simulink model "receiver_overall_reset"  (Simulink 7.5)
settings: Solver=FixedStepDiscrete  SolverMode=SingleTasking  StartTime=0.0  StopTime=(length(simin.signals.values)-1)/Fs  FixedStep=1  RelTol=1e-3
undefined symbols (not defined in the file): Fs
libraries: xbsIndex_r4 x962
(part 5 of 9)

== system receiver_overall_reset/Receiver/Sym-Chooser/2-10/Corr0/Corr ==
  In1 : Inport
  AddSub{,1..6} (7 alike) : xbsIndex_r4/AddSub  mode=Addition  use_carryin=off  use_carryout=off  en=off  latency=0  precision=Full  arith_type=Unsigned  n_bits=16  bin_pt=14  quantization=Truncate  overflow=Wrap  dbl_ovrd=off  use_behavioral_HDL=off  hw_selection=Fabric  pipelined=off  block_type=addsub
      AddSub settings: xl_area=[2 0 0 3 0 0 0]  block_version=12.1
      AddSub1 settings: xl_area=[2 0 0 3 0 0 0]  block_version=12.1
      AddSub2 settings: xl_area=[3 0 0 4 0 0 0]  block_version=12.1
      AddSub3 settings: xl_area=[3 0 0 5 0 0 0]  block_version=12.1
      AddSub4 settings: xl_area=[2 0 0 3 0 0 0]  block_version=12.1
      AddSub5 settings: xl_area=[2 0 0 3 0 0 0]  block_version=12.1
      AddSub6 settings: xl_area=[3 0 0 4 0 0 0]  block_version=12.1
  LUT{0..7} (8 alike) : xbsIndex_r4/ROM  depth=16  initVector=[0,1,1,2,1,2,2,3,1,2,2,3,2,3,3,4]  distributed_mem=Distributed memory  rst=off  init_reg=0  en=off  latency=0  arith_type=Unsigned  n_bits=3  bin_pt=0  dbl_ovrd=off  optimize=Area  use_rpm=on  block_type=sprom
      settings: xl_area=[0 0 1 0 0 0 0]  block_version=12.1
  Slice0 : xbsIndex_r4/Slice  nbits=4  boolean_output=off  mode=Lower Bit Location + Width  bit1=0  base1=MSB of Input  bit0=0  base0=LSB of Input  dbl_ovrd=off  block_type=slice
      settings: block_version=12.1
  Slice1 : xbsIndex_r4/Slice  nbits=4  boolean_output=off  mode=Lower Bit Location + Width  bit1=-4  base1=MSB of Input  bit0=4  base0=LSB of Input  dbl_ovrd=off  block_type=slice
      settings: block_version=12.1
  Slice2 : xbsIndex_r4/Slice  nbits=4  boolean_output=off  mode=Lower Bit Location + Width  bit1=-8  base1=MSB of Input  bit0=8  base0=LSB of Input  dbl_ovrd=off  block_type=slice
      settings: block_version=12.1
  Slice3 : xbsIndex_r4/Slice  nbits=4  boolean_output=off  mode=Lower Bit Location + Width  bit1=-12  base1=MSB of Input  bit0=12  base0=LSB of Input  dbl_ovrd=off  block_type=slice
      settings: block_version=12.1
  Slice4 : xbsIndex_r4/Slice  nbits=4  boolean_output=off  mode=Lower Bit Location + Width  bit1=0  base1=LSB of Input  bit0=16  base0=LSB of Input  dbl_ovrd=off  block_type=slice
      settings: block_version=12.1
  Slice5 : xbsIndex_r4/Slice  nbits=4  boolean_output=off  mode=Lower Bit Location + Width  bit1=0  base1=LSB of Input  bit0=20  base0=LSB of Input  dbl_ovrd=off  block_type=slice
      settings: block_version=12.1
  Slice6 : xbsIndex_r4/Slice  nbits=4  boolean_output=off  mode=Lower Bit Location + Width  bit1=0  base1=LSB of Input  bit0=24  base0=LSB of Input  dbl_ovrd=off  block_type=slice
      settings: block_version=12.1
  Slice7 : xbsIndex_r4/Slice  nbits=4  boolean_output=off  mode=Lower Bit Location + Width  bit1=0  base1=LSB of Input  bit0=28  base0=LSB of Input  dbl_ovrd=off  block_type=slice
      settings: block_version=12.1
  Out2 : Outport
  wires:
  In1/1 -> Slice0/1, Slice1/1, Slice2/1, Slice7/1, Slice6/1, Slice3/1, Slice4/1, Slice5/1
  Slice0/1 -> LUT0/1
  Slice3/1 -> LUT3/1
  Slice2/1 -> LUT2/1
  Slice1/1 -> LUT1/1
  LUT0/1 -> AddSub/1
  LUT1/1 -> AddSub/2
  LUT2/1 -> AddSub1/1
  LUT3/1 -> AddSub1/2
  AddSub1/1 -> AddSub2/2
  AddSub/1 -> AddSub2/1
  AddSub3/1 -> Out2/1
  Slice4/1 -> LUT4/1
  Slice7/1 -> LUT7/1
  Slice6/1 -> LUT6/1
  Slice5/1 -> LUT5/1
  LUT4/1 -> AddSub4/1
  LUT5/1 -> AddSub4/2
  LUT6/1 -> AddSub5/1
  LUT7/1 -> AddSub5/2
  AddSub5/1 -> AddSub6/2
  AddSub4/1 -> AddSub6/1
  AddSub2/1 -> AddSub3/1
  AddSub6/1 -> AddSub3/2

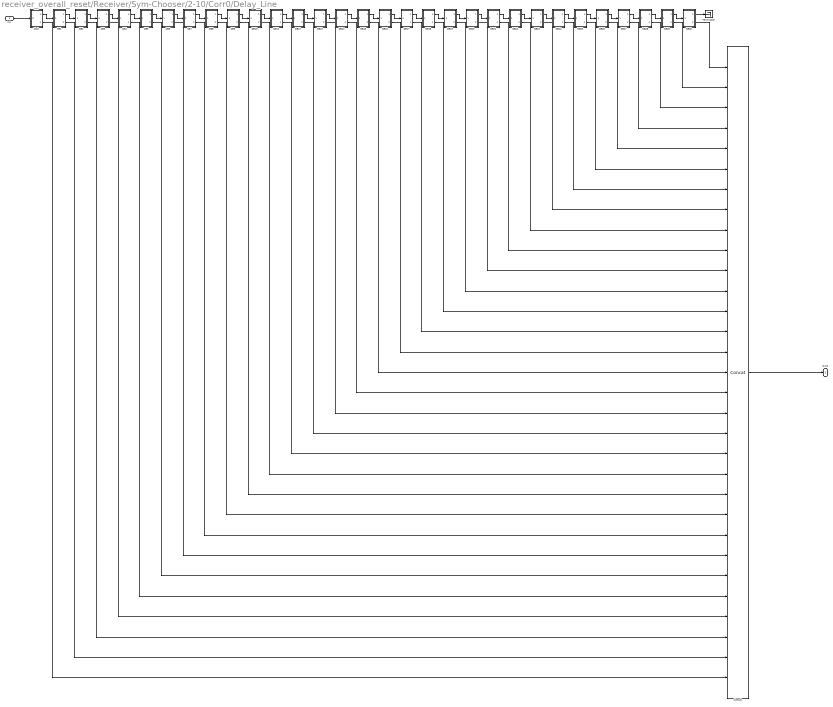
== system receiver_overall_reset/Receiver/Sym-Chooser/2-10/Corr0/Delay_Line ==
  In1 : Inport
  1to2 : Subsystem
  Concat : xbsIndex_r4/Concat  num_inputs=31  dbl_ovrd=off  block_type=concat
      settings: block_version=12.1
  DE1 : Subsystem
      mask Display: disp('z^{-1}','texmode','on')
  DE10 : Subsystem
      mask Display: disp('z^{-1}','texmode','on')
  DE11 : Subsystem
      mask Display: disp('z^{-1}','texmode','on')
  DE12 : Subsystem
      mask Display: disp('z^{-1}','texmode','on')
  DE13 : Subsystem
      mask Display: disp('z^{-1}','texmode','on')
  DE14 : Subsystem
      mask Display: disp('z^{-1}','texmode','on')
  DE15 : Subsystem
      mask Display: disp('z^{-1}','texmode','on')
  DE16 : Subsystem
      mask Display: disp('z^{-1}','texmode','on')
  DE17 : Subsystem
      mask Display: disp('z^{-1}','texmode','on')
  DE18 : Subsystem
      mask Display: disp('z^{-1}','texmode','on')
  DE19 : Subsystem
      mask Display: disp('z^{-1}','texmode','on')
  DE2 : Subsystem
      mask Display: disp('z^{-1}','texmode','on')
  DE20 : Subsystem
      mask Display: disp('z^{-1}','texmode','on')
  DE21 : Subsystem
      mask Display: disp('z^{-1}','texmode','on')
  DE22 : Subsystem
      mask Display: disp('z^{-1}','texmode','on')
  DE23 : Subsystem
      mask Display: disp('z^{-1}','texmode','on')
  DE24 : Subsystem
      mask Display: disp('z^{-1}','texmode','on')
  DE25 : Subsystem
      mask Display: disp('z^{-1}','texmode','on')
  DE26 : Subsystem
      mask Display: disp('z^{-1}','texmode','on')
  DE27 : Subsystem
      mask Display: disp('z^{-1}','texmode','on')
  DE28 : Subsystem
      mask Display: disp('z^{-1}','texmode','on')
  DE29 : Subsystem
      mask Display: disp('z^{-1}','texmode','on')
  DE3 : Subsystem
      mask Display: disp('z^{-1}','texmode','on')
  DE30 : Subsystem
      mask Display: disp('z^{-1}','texmode','on')
  DE4 : Subsystem
      mask Display: disp('z^{-1}','texmode','on')
  DE5 : Subsystem
      mask Display: disp('z^{-1}','texmode','on')
  DE6 : Subsystem
      mask Display: disp('z^{-1}','texmode','on')
  DE7 : Subsystem
      mask Display: disp('z^{-1}','texmode','on')
  DE8 : Subsystem
      mask Display: disp('z^{-1}','texmode','on')
  DE9 : Subsystem
      mask Display: disp('z^{-1}','texmode','on')
  Terminator : Terminator
  Out2 : Outport
  wires:
  Concat/1 -> Out2/1
  In1/1 -> 1to2/1(In)
  1to2/1(Out1) -> DE1/1(In1)
  DE30/1(Out1) -> Terminator/1
  1to2/2(Out2) -> Concat/31
  DE1/2(Out2) -> Concat/30
  DE2/2(Out2) -> Concat/29
  DE3/2(Out2) -> Concat/28
  DE4/2(Out2) -> Concat/27
  DE5/2(Out2) -> Concat/26
  DE6/2(Out2) -> Concat/25
  DE7/2(Out2) -> Concat/24
  DE8/2(Out2) -> Concat/23
  DE9/2(Out2) -> Concat/22
  DE10/2(Out2) -> Concat/21
  DE11/2(Out2) -> Concat/20
  DE12/2(Out2) -> Concat/19
  DE13/2(Out2) -> Concat/18
  DE14/2(Out2) -> Concat/17
  DE15/2(Out2) -> Concat/16
  DE16/2(Out2) -> Concat/15
  DE17/2(Out2) -> Concat/14
  DE18/2(Out2) -> Concat/13
  DE19/2(Out2) -> Concat/12
  DE20/2(Out2) -> Concat/11
  DE21/2(Out2) -> Concat/10
  DE22/2(Out2) -> Concat/9
  DE23/2(Out2) -> Concat/8
  DE24/2(Out2) -> Concat/7
  DE25/2(Out2) -> Concat/6
  DE26/2(Out2) -> Concat/5
  DE27/2(Out2) -> Concat/4
  DE28/2(Out2) -> Concat/3
  DE29/2(Out2) -> Concat/2
  DE30/2(Out2) -> Concat/1
  DE2/1(Out1) -> DE3/1(In1)
  DE3/1(Out1) -> DE4/1(In1)
  DE4/1(Out1) -> DE5/1(In1)
  DE5/1(Out1) -> DE6/1(In1)
  DE6/1(Out1) -> DE7/1(In1)
  DE7/1(Out1) -> DE8/1(In1)
  DE8/1(Out1) -> DE9/1(In1)
  DE9/1(Out1) -> DE10/1(In1)
  DE10/1(Out1) -> DE11/1(In1)
  DE11/1(Out1) -> DE12/1(In1)
  DE12/1(Out1) -> DE13/1(In1)
  DE13/1(Out1) -> DE14/1(In1)
  DE14/1(Out1) -> DE15/1(In1)
  DE15/1(Out1) -> DE16/1(In1)
  DE16/1(Out1) -> DE17/1(In1)
  DE17/1(Out1) -> DE18/1(In1)
  DE18/1(Out1) -> DE19/1(In1)
  DE19/1(Out1) -> DE20/1(In1)
  DE20/1(Out1) -> DE21/1(In1)
  DE21/1(Out1) -> DE22/1(In1)
  DE22/1(Out1) -> DE23/1(In1)
  DE23/1(Out1) -> DE24/1(In1)
  DE24/1(Out1) -> DE25/1(In1)
  DE25/1(Out1) -> DE26/1(In1)
  DE26/1(Out1) -> DE27/1(In1)
  DE27/1(Out1) -> DE28/1(In1)
  DE28/1(Out1) -> DE29/1(In1)
  DE29/1(Out1) -> DE30/1(In1)
  DE1/1(Out1) -> DE2/1(In1)

== system receiver_overall_reset/Receiver/Sym-Chooser/3-11/Corr0/Corr ==
  In1 : Inport
  AddSub{,1..6} (7 alike) : xbsIndex_r4/AddSub  mode=Addition  use_carryin=off  use_carryout=off  en=off  latency=0  precision=Full  arith_type=Unsigned  n_bits=16  bin_pt=14  quantization=Truncate  overflow=Wrap  dbl_ovrd=off  use_behavioral_HDL=off  hw_selection=Fabric  pipelined=off  block_type=addsub
      AddSub settings: xl_area=[2 0 0 3 0 0 0]  block_version=12.1
      AddSub1 settings: xl_area=[2 0 0 3 0 0 0]  block_version=12.1
      AddSub2 settings: xl_area=[3 0 0 4 0 0 0]  block_version=12.1
      AddSub3 settings: xl_area=[3 0 0 5 0 0 0]  block_version=12.1
      AddSub4 settings: xl_area=[2 0 0 3 0 0 0]  block_version=12.1
      AddSub5 settings: xl_area=[2 0 0 3 0 0 0]  block_version=12.1
      AddSub6 settings: xl_area=[3 0 0 4 0 0 0]  block_version=12.1
  LUT{0..7} (8 alike) : xbsIndex_r4/ROM  depth=16  initVector=[0,1,1,2,1,2,2,3,1,2,2,3,2,3,3,4]  distributed_mem=Distributed memory  rst=off  init_reg=0  en=off  latency=0  arith_type=Unsigned  n_bits=3  bin_pt=0  dbl_ovrd=off  optimize=Area  use_rpm=on  block_type=sprom
      settings: xl_area=[0 0 1 0 0 0 0]  block_version=12.1
  Slice0 : xbsIndex_r4/Slice  nbits=4  boolean_output=off  mode=Lower Bit Location + Width  bit1=0  base1=MSB of Input  bit0=0  base0=LSB of Input  dbl_ovrd=off  block_type=slice
      settings: block_version=12.1
  Slice1 : xbsIndex_r4/Slice  nbits=4  boolean_output=off  mode=Lower Bit Location + Width  bit1=-4  base1=MSB of Input  bit0=4  base0=LSB of Input  dbl_ovrd=off  block_type=slice
      settings: block_version=12.1
  Slice2 : xbsIndex_r4/Slice  nbits=4  boolean_output=off  mode=Lower Bit Location + Width  bit1=-8  base1=MSB of Input  bit0=8  base0=LSB of Input  dbl_ovrd=off  block_type=slice
      settings: block_version=12.1
  Slice3 : xbsIndex_r4/Slice  nbits=4  boolean_output=off  mode=Lower Bit Location + Width  bit1=-12  base1=MSB of Input  bit0=12  base0=LSB of Input  dbl_ovrd=off  block_type=slice
      settings: block_version=12.1
  Slice4 : xbsIndex_r4/Slice  nbits=4  boolean_output=off  mode=Lower Bit Location + Width  bit1=0  base1=LSB of Input  bit0=16  base0=LSB of Input  dbl_ovrd=off  block_type=slice
      settings: block_version=12.1
  Slice5 : xbsIndex_r4/Slice  nbits=4  boolean_output=off  mode=Lower Bit Location + Width  bit1=0  base1=LSB of Input  bit0=20  base0=LSB of Input  dbl_ovrd=off  block_type=slice
      settings: block_version=12.1
  Slice6 : xbsIndex_r4/Slice  nbits=4  boolean_output=off  mode=Lower Bit Location + Width  bit1=0  base1=LSB of Input  bit0=24  base0=LSB of Input  dbl_ovrd=off  block_type=slice
      settings: block_version=12.1
  Slice7 : xbsIndex_r4/Slice  nbits=4  boolean_output=off  mode=Lower Bit Location + Width  bit1=0  base1=LSB of Input  bit0=28  base0=LSB of Input  dbl_ovrd=off  block_type=slice
      settings: block_version=12.1
  Out2 : Outport
  wires:
  In1/1 -> Slice0/1, Slice1/1, Slice2/1, Slice7/1, Slice6/1, Slice3/1, Slice4/1, Slice5/1
  Slice0/1 -> LUT0/1
  Slice3/1 -> LUT3/1
  Slice2/1 -> LUT2/1
  Slice1/1 -> LUT1/1
  LUT0/1 -> AddSub/1
  LUT1/1 -> AddSub/2
  LUT2/1 -> AddSub1/1
  LUT3/1 -> AddSub1/2
  AddSub1/1 -> AddSub2/2
  AddSub/1 -> AddSub2/1
  AddSub3/1 -> Out2/1
  Slice4/1 -> LUT4/1
  Slice7/1 -> LUT7/1
  Slice6/1 -> LUT6/1
  Slice5/1 -> LUT5/1
  LUT4/1 -> AddSub4/1
  LUT5/1 -> AddSub4/2
  LUT6/1 -> AddSub5/1
  LUT7/1 -> AddSub5/2
  AddSub5/1 -> AddSub6/2
  AddSub4/1 -> AddSub6/1
  AddSub2/1 -> AddSub3/1
  AddSub6/1 -> AddSub3/2

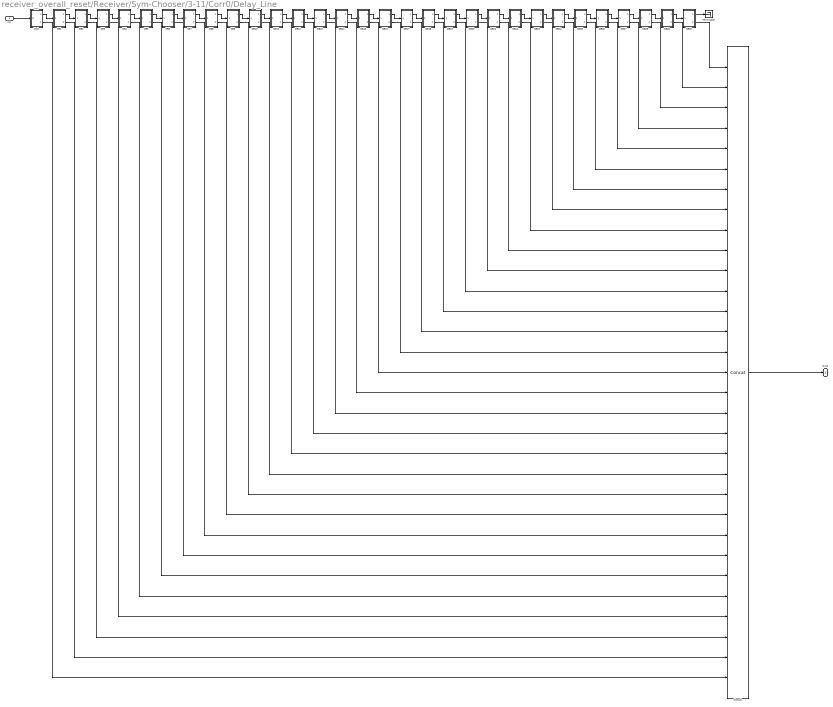
== system receiver_overall_reset/Receiver/Sym-Chooser/3-11/Corr0/Delay_Line ==
  In1 : Inport
  1to2 : Subsystem
  Concat : xbsIndex_r4/Concat  num_inputs=31  dbl_ovrd=off  block_type=concat
      settings: block_version=12.1
  DE1 : Subsystem
      mask Display: disp('z^{-1}','texmode','on')
  DE10 : Subsystem
      mask Display: disp('z^{-1}','texmode','on')
  DE11 : Subsystem
      mask Display: disp('z^{-1}','texmode','on')
  DE12 : Subsystem
      mask Display: disp('z^{-1}','texmode','on')
  DE13 : Subsystem
      mask Display: disp('z^{-1}','texmode','on')
  DE14 : Subsystem
      mask Display: disp('z^{-1}','texmode','on')
  DE15 : Subsystem
      mask Display: disp('z^{-1}','texmode','on')
  DE16 : Subsystem
      mask Display: disp('z^{-1}','texmode','on')
  DE17 : Subsystem
      mask Display: disp('z^{-1}','texmode','on')
  DE18 : Subsystem
      mask Display: disp('z^{-1}','texmode','on')
  DE19 : Subsystem
      mask Display: disp('z^{-1}','texmode','on')
  DE2 : Subsystem
      mask Display: disp('z^{-1}','texmode','on')
  DE20 : Subsystem
      mask Display: disp('z^{-1}','texmode','on')
  DE21 : Subsystem
      mask Display: disp('z^{-1}','texmode','on')
  DE22 : Subsystem
      mask Display: disp('z^{-1}','texmode','on')
  DE23 : Subsystem
      mask Display: disp('z^{-1}','texmode','on')
  DE24 : Subsystem
      mask Display: disp('z^{-1}','texmode','on')
  DE25 : Subsystem
      mask Display: disp('z^{-1}','texmode','on')
  DE26 : Subsystem
      mask Display: disp('z^{-1}','texmode','on')
  DE27 : Subsystem
      mask Display: disp('z^{-1}','texmode','on')
  DE28 : Subsystem
      mask Display: disp('z^{-1}','texmode','on')
  DE29 : Subsystem
      mask Display: disp('z^{-1}','texmode','on')
  DE3 : Subsystem
      mask Display: disp('z^{-1}','texmode','on')
  DE30 : Subsystem
      mask Display: disp('z^{-1}','texmode','on')
  DE4 : Subsystem
      mask Display: disp('z^{-1}','texmode','on')
  DE5 : Subsystem
      mask Display: disp('z^{-1}','texmode','on')
  DE6 : Subsystem
      mask Display: disp('z^{-1}','texmode','on')
  DE7 : Subsystem
      mask Display: disp('z^{-1}','texmode','on')
  DE8 : Subsystem
      mask Display: disp('z^{-1}','texmode','on')
  DE9 : Subsystem
      mask Display: disp('z^{-1}','texmode','on')
  Terminator : Terminator
  Out2 : Outport
  wires:
  Concat/1 -> Out2/1
  In1/1 -> 1to2/1(In)
  1to2/1(Out1) -> DE1/1(In1)
  DE30/1(Out1) -> Terminator/1
  1to2/2(Out2) -> Concat/31
  DE1/2(Out2) -> Concat/30
  DE2/2(Out2) -> Concat/29
  DE3/2(Out2) -> Concat/28
  DE4/2(Out2) -> Concat/27
  DE5/2(Out2) -> Concat/26
  DE6/2(Out2) -> Concat/25
  DE7/2(Out2) -> Concat/24
  DE8/2(Out2) -> Concat/23
  DE9/2(Out2) -> Concat/22
  DE10/2(Out2) -> Concat/21
  DE11/2(Out2) -> Concat/20
  DE12/2(Out2) -> Concat/19
  DE13/2(Out2) -> Concat/18
  DE14/2(Out2) -> Concat/17
  DE15/2(Out2) -> Concat/16
  DE16/2(Out2) -> Concat/15
  DE17/2(Out2) -> Concat/14
  DE18/2(Out2) -> Concat/13
  DE19/2(Out2) -> Concat/12
  DE20/2(Out2) -> Concat/11
  DE21/2(Out2) -> Concat/10
  DE22/2(Out2) -> Concat/9
  DE23/2(Out2) -> Concat/8
  DE24/2(Out2) -> Concat/7
  DE25/2(Out2) -> Concat/6
  DE26/2(Out2) -> Concat/5
  DE27/2(Out2) -> Concat/4
  DE28/2(Out2) -> Concat/3
  DE29/2(Out2) -> Concat/2
  DE30/2(Out2) -> Concat/1
  DE2/1(Out1) -> DE3/1(In1)
  DE3/1(Out1) -> DE4/1(In1)
  DE4/1(Out1) -> DE5/1(In1)
  DE5/1(Out1) -> DE6/1(In1)
  DE6/1(Out1) -> DE7/1(In1)
  DE7/1(Out1) -> DE8/1(In1)
  DE8/1(Out1) -> DE9/1(In1)
  DE9/1(Out1) -> DE10/1(In1)
  DE10/1(Out1) -> DE11/1(In1)
  DE11/1(Out1) -> DE12/1(In1)
  DE12/1(Out1) -> DE13/1(In1)
  DE13/1(Out1) -> DE14/1(In1)
  DE14/1(Out1) -> DE15/1(In1)
  DE15/1(Out1) -> DE16/1(In1)
  DE16/1(Out1) -> DE17/1(In1)
  DE17/1(Out1) -> DE18/1(In1)
  DE18/1(Out1) -> DE19/1(In1)
  DE19/1(Out1) -> DE20/1(In1)
  DE20/1(Out1) -> DE21/1(In1)
  DE21/1(Out1) -> DE22/1(In1)
  DE22/1(Out1) -> DE23/1(In1)
  DE23/1(Out1) -> DE24/1(In1)
  DE24/1(Out1) -> DE25/1(In1)
  DE25/1(Out1) -> DE26/1(In1)
  DE26/1(Out1) -> DE27/1(In1)
  DE27/1(Out1) -> DE28/1(In1)
  DE28/1(Out1) -> DE29/1(In1)
  DE29/1(Out1) -> DE30/1(In1)
  DE1/1(Out1) -> DE2/1(In1)

== system receiver_overall_reset/Receiver/Sym-Chooser/4-12/Corr0/Corr ==
  In1 : Inport
  AddSub{,1..6} (7 alike) : xbsIndex_r4/AddSub  mode=Addition  use_carryin=off  use_carryout=off  en=off  latency=0  precision=Full  arith_type=Unsigned  n_bits=16  bin_pt=14  quantization=Truncate  overflow=Wrap  dbl_ovrd=off  use_behavioral_HDL=off  hw_selection=Fabric  pipelined=off  block_type=addsub
      AddSub settings: xl_area=[2 0 0 3 0 0 0]  block_version=12.1
      AddSub1 settings: xl_area=[2 0 0 3 0 0 0]  block_version=12.1
      AddSub2 settings: xl_area=[3 0 0 4 0 0 0]  block_version=12.1
      AddSub3 settings: xl_area=[3 0 0 5 0 0 0]  block_version=12.1
      AddSub4 settings: xl_area=[2 0 0 3 0 0 0]  block_version=12.1
      AddSub5 settings: xl_area=[2 0 0 3 0 0 0]  block_version=12.1
      AddSub6 settings: xl_area=[3 0 0 4 0 0 0]  block_version=12.1
  LUT{0..7} (8 alike) : xbsIndex_r4/ROM  depth=16  initVector=[0,1,1,2,1,2,2,3,1,2,2,3,2,3,3,4]  distributed_mem=Distributed memory  rst=off  init_reg=0  en=off  latency=0  arith_type=Unsigned  n_bits=3  bin_pt=0  dbl_ovrd=off  optimize=Area  use_rpm=on  block_type=sprom
      settings: xl_area=[0 0 1 0 0 0 0]  block_version=12.1
  Slice0 : xbsIndex_r4/Slice  nbits=4  boolean_output=off  mode=Lower Bit Location + Width  bit1=0  base1=MSB of Input  bit0=0  base0=LSB of Input  dbl_ovrd=off  block_type=slice
      settings: block_version=12.1
  Slice1 : xbsIndex_r4/Slice  nbits=4  boolean_output=off  mode=Lower Bit Location + Width  bit1=-4  base1=MSB of Input  bit0=4  base0=LSB of Input  dbl_ovrd=off  block_type=slice
      settings: block_version=12.1
  Slice2 : xbsIndex_r4/Slice  nbits=4  boolean_output=off  mode=Lower Bit Location + Width  bit1=-8  base1=MSB of Input  bit0=8  base0=LSB of Input  dbl_ovrd=off  block_type=slice
      settings: block_version=12.1
  Slice3 : xbsIndex_r4/Slice  nbits=4  boolean_output=off  mode=Lower Bit Location + Width  bit1=-12  base1=MSB of Input  bit0=12  base0=LSB of Input  dbl_ovrd=off  block_type=slice
      settings: block_version=12.1
  Slice4 : xbsIndex_r4/Slice  nbits=4  boolean_output=off  mode=Lower Bit Location + Width  bit1=0  base1=LSB of Input  bit0=16  base0=LSB of Input  dbl_ovrd=off  block_type=slice
      settings: block_version=12.1
  Slice5 : xbsIndex_r4/Slice  nbits=4  boolean_output=off  mode=Lower Bit Location + Width  bit1=0  base1=LSB of Input  bit0=20  base0=LSB of Input  dbl_ovrd=off  block_type=slice
      settings: block_version=12.1
  Slice6 : xbsIndex_r4/Slice  nbits=4  boolean_output=off  mode=Lower Bit Location + Width  bit1=0  base1=LSB of Input  bit0=24  base0=LSB of Input  dbl_ovrd=off  block_type=slice
      settings: block_version=12.1
  Slice7 : xbsIndex_r4/Slice  nbits=4  boolean_output=off  mode=Lower Bit Location + Width  bit1=0  base1=LSB of Input  bit0=28  base0=LSB of Input  dbl_ovrd=off  block_type=slice
      settings: block_version=12.1
  Out2 : Outport
  wires:
  In1/1 -> Slice0/1, Slice1/1, Slice2/1, Slice7/1, Slice6/1, Slice3/1, Slice4/1, Slice5/1
  Slice0/1 -> LUT0/1
  Slice3/1 -> LUT3/1
  Slice2/1 -> LUT2/1
  Slice1/1 -> LUT1/1
  LUT0/1 -> AddSub/1
  LUT1/1 -> AddSub/2
  LUT2/1 -> AddSub1/1
  LUT3/1 -> AddSub1/2
  AddSub1/1 -> AddSub2/2
  AddSub/1 -> AddSub2/1
  AddSub3/1 -> Out2/1
  Slice4/1 -> LUT4/1
  Slice7/1 -> LUT7/1
  Slice6/1 -> LUT6/1
  Slice5/1 -> LUT5/1
  LUT4/1 -> AddSub4/1
  LUT5/1 -> AddSub4/2
  LUT6/1 -> AddSub5/1
  LUT7/1 -> AddSub5/2
  AddSub5/1 -> AddSub6/2
  AddSub4/1 -> AddSub6/1
  AddSub2/1 -> AddSub3/1
  AddSub6/1 -> AddSub3/2

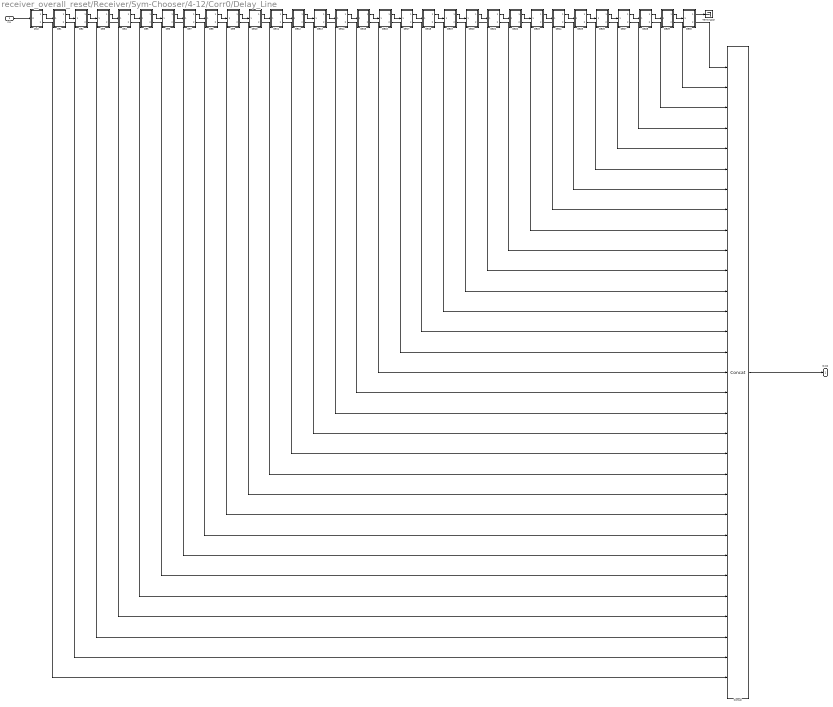
== system receiver_overall_reset/Receiver/Sym-Chooser/4-12/Corr0/Delay_Line ==
  In1 : Inport
  1to2 : Subsystem
  Concat : xbsIndex_r4/Concat  num_inputs=31  dbl_ovrd=off  block_type=concat
      settings: block_version=12.1
  DE1 : Subsystem
      mask Display: disp('z^{-1}','texmode','on')
  DE10 : Subsystem
      mask Display: disp('z^{-1}','texmode','on')
  DE11 : Subsystem
      mask Display: disp('z^{-1}','texmode','on')
  DE12 : Subsystem
      mask Display: disp('z^{-1}','texmode','on')
  DE13 : Subsystem
      mask Display: disp('z^{-1}','texmode','on')
  DE14 : Subsystem
      mask Display: disp('z^{-1}','texmode','on')
  DE15 : Subsystem
      mask Display: disp('z^{-1}','texmode','on')
  DE16 : Subsystem
      mask Display: disp('z^{-1}','texmode','on')
  DE17 : Subsystem
      mask Display: disp('z^{-1}','texmode','on')
  DE18 : Subsystem
      mask Display: disp('z^{-1}','texmode','on')
  DE19 : Subsystem
      mask Display: disp('z^{-1}','texmode','on')
  DE2 : Subsystem
      mask Display: disp('z^{-1}','texmode','on')
  DE20 : Subsystem
      mask Display: disp('z^{-1}','texmode','on')
  DE21 : Subsystem
      mask Display: disp('z^{-1}','texmode','on')
  DE22 : Subsystem
      mask Display: disp('z^{-1}','texmode','on')
  DE23 : Subsystem
      mask Display: disp('z^{-1}','texmode','on')
  DE24 : Subsystem
      mask Display: disp('z^{-1}','texmode','on')
  DE25 : Subsystem
      mask Display: disp('z^{-1}','texmode','on')
  DE26 : Subsystem
      mask Display: disp('z^{-1}','texmode','on')
  DE27 : Subsystem
      mask Display: disp('z^{-1}','texmode','on')
  DE28 : Subsystem
      mask Display: disp('z^{-1}','texmode','on')
  DE29 : Subsystem
      mask Display: disp('z^{-1}','texmode','on')
  DE3 : Subsystem
      mask Display: disp('z^{-1}','texmode','on')
  DE30 : Subsystem
      mask Display: disp('z^{-1}','texmode','on')
  DE4 : Subsystem
      mask Display: disp('z^{-1}','texmode','on')
  DE5 : Subsystem
      mask Display: disp('z^{-1}','texmode','on')
  DE6 : Subsystem
      mask Display: disp('z^{-1}','texmode','on')
  DE7 : Subsystem
      mask Display: disp('z^{-1}','texmode','on')
  DE8 : Subsystem
      mask Display: disp('z^{-1}','texmode','on')
  DE9 : Subsystem
      mask Display: disp('z^{-1}','texmode','on')
  Terminator : Terminator
  Out2 : Outport
  wires:
  Concat/1 -> Out2/1
  In1/1 -> 1to2/1(In)
  1to2/1(Out1) -> DE1/1(In1)
  DE30/1(Out1) -> Terminator/1
  1to2/2(Out2) -> Concat/31
  DE1/2(Out2) -> Concat/30
  DE2/2(Out2) -> Concat/29
  DE3/2(Out2) -> Concat/28
  DE4/2(Out2) -> Concat/27
  DE5/2(Out2) -> Concat/26
  DE6/2(Out2) -> Concat/25
  DE7/2(Out2) -> Concat/24
  DE8/2(Out2) -> Concat/23
  DE9/2(Out2) -> Concat/22
  DE10/2(Out2) -> Concat/21
  DE11/2(Out2) -> Concat/20
  DE12/2(Out2) -> Concat/19
  DE13/2(Out2) -> Concat/18
  DE14/2(Out2) -> Concat/17
  DE15/2(Out2) -> Concat/16
  DE16/2(Out2) -> Concat/15
  DE17/2(Out2) -> Concat/14
  DE18/2(Out2) -> Concat/13
  DE19/2(Out2) -> Concat/12
  DE20/2(Out2) -> Concat/11
  DE21/2(Out2) -> Concat/10
  DE22/2(Out2) -> Concat/9
  DE23/2(Out2) -> Concat/8
  DE24/2(Out2) -> Concat/7
  DE25/2(Out2) -> Concat/6
  DE26/2(Out2) -> Concat/5
  DE27/2(Out2) -> Concat/4
  DE28/2(Out2) -> Concat/3
  DE29/2(Out2) -> Concat/2
  DE30/2(Out2) -> Concat/1
  DE2/1(Out1) -> DE3/1(In1)
  DE3/1(Out1) -> DE4/1(In1)
  DE4/1(Out1) -> DE5/1(In1)
  DE5/1(Out1) -> DE6/1(In1)
  DE6/1(Out1) -> DE7/1(In1)
  DE7/1(Out1) -> DE8/1(In1)
  DE8/1(Out1) -> DE9/1(In1)
  DE9/1(Out1) -> DE10/1(In1)
  DE10/1(Out1) -> DE11/1(In1)
  DE11/1(Out1) -> DE12/1(In1)
  DE12/1(Out1) -> DE13/1(In1)
  DE13/1(Out1) -> DE14/1(In1)
  DE14/1(Out1) -> DE15/1(In1)
  DE15/1(Out1) -> DE16/1(In1)
  DE16/1(Out1) -> DE17/1(In1)
  DE17/1(Out1) -> DE18/1(In1)
  DE18/1(Out1) -> DE19/1(In1)
  DE19/1(Out1) -> DE20/1(In1)
  DE20/1(Out1) -> DE21/1(In1)
  DE21/1(Out1) -> DE22/1(In1)
  DE22/1(Out1) -> DE23/1(In1)
  DE23/1(Out1) -> DE24/1(In1)
  DE24/1(Out1) -> DE25/1(In1)
  DE25/1(Out1) -> DE26/1(In1)
  DE26/1(Out1) -> DE27/1(In1)
  DE27/1(Out1) -> DE28/1(In1)
  DE28/1(Out1) -> DE29/1(In1)
  DE29/1(Out1) -> DE30/1(In1)
  DE1/1(Out1) -> DE2/1(In1)

== system receiver_overall_reset/Receiver/Sym-Chooser/5-13/Corr0/Corr ==
  In1 : Inport
  AddSub{,1..6} (7 alike) : xbsIndex_r4/AddSub  mode=Addition  use_carryin=off  use_carryout=off  en=off  latency=0  precision=Full  arith_type=Unsigned  n_bits=16  bin_pt=14  quantization=Truncate  overflow=Wrap  dbl_ovrd=off  use_behavioral_HDL=off  hw_selection=Fabric  pipelined=off  block_type=addsub
      AddSub settings: xl_area=[2 0 0 3 0 0 0]  block_version=12.1
      AddSub1 settings: xl_area=[2 0 0 3 0 0 0]  block_version=12.1
      AddSub2 settings: xl_area=[3 0 0 4 0 0 0]  block_version=12.1
      AddSub3 settings: xl_area=[3 0 0 5 0 0 0]  block_version=12.1
      AddSub4 settings: xl_area=[2 0 0 3 0 0 0]  block_version=12.1
      AddSub5 settings: xl_area=[2 0 0 3 0 0 0]  block_version=12.1
      AddSub6 settings: xl_area=[3 0 0 4 0 0 0]  block_version=12.1
  LUT{0..7} (8 alike) : xbsIndex_r4/ROM  depth=16  initVector=[0,1,1,2,1,2,2,3,1,2,2,3,2,3,3,4]  distributed_mem=Distributed memory  rst=off  init_reg=0  en=off  latency=0  arith_type=Unsigned  n_bits=3  bin_pt=0  dbl_ovrd=off  optimize=Area  use_rpm=on  block_type=sprom
      settings: xl_area=[0 0 1 0 0 0 0]  block_version=12.1
  Slice0 : xbsIndex_r4/Slice  nbits=4  boolean_output=off  mode=Lower Bit Location + Width  bit1=0  base1=MSB of Input  bit0=0  base0=LSB of Input  dbl_ovrd=off  block_type=slice
      settings: block_version=12.1
  Slice1 : xbsIndex_r4/Slice  nbits=4  boolean_output=off  mode=Lower Bit Location + Width  bit1=-4  base1=MSB of Input  bit0=4  base0=LSB of Input  dbl_ovrd=off  block_type=slice
      settings: block_version=12.1
  Slice2 : xbsIndex_r4/Slice  nbits=4  boolean_output=off  mode=Lower Bit Location + Width  bit1=-8  base1=MSB of Input  bit0=8  base0=LSB of Input  dbl_ovrd=off  block_type=slice
      settings: block_version=12.1
  Slice3 : xbsIndex_r4/Slice  nbits=4  boolean_output=off  mode=Lower Bit Location + Width  bit1=-12  base1=MSB of Input  bit0=12  base0=LSB of Input  dbl_ovrd=off  block_type=slice
      settings: block_version=12.1
  Slice4 : xbsIndex_r4/Slice  nbits=4  boolean_output=off  mode=Lower Bit Location + Width  bit1=0  base1=LSB of Input  bit0=16  base0=LSB of Input  dbl_ovrd=off  block_type=slice
      settings: block_version=12.1
  Slice5 : xbsIndex_r4/Slice  nbits=4  boolean_output=off  mode=Lower Bit Location + Width  bit1=0  base1=LSB of Input  bit0=20  base0=LSB of Input  dbl_ovrd=off  block_type=slice
      settings: block_version=12.1
  Slice6 : xbsIndex_r4/Slice  nbits=4  boolean_output=off  mode=Lower Bit Location + Width  bit1=0  base1=LSB of Input  bit0=24  base0=LSB of Input  dbl_ovrd=off  block_type=slice
      settings: block_version=12.1
  Slice7 : xbsIndex_r4/Slice  nbits=4  boolean_output=off  mode=Lower Bit Location + Width  bit1=0  base1=LSB of Input  bit0=28  base0=LSB of Input  dbl_ovrd=off  block_type=slice
      settings: block_version=12.1
  Out2 : Outport
  wires:
  In1/1 -> Slice0/1, Slice1/1, Slice2/1, Slice7/1, Slice6/1, Slice3/1, Slice4/1, Slice5/1
  Slice0/1 -> LUT0/1
  Slice3/1 -> LUT3/1
  Slice2/1 -> LUT2/1
  Slice1/1 -> LUT1/1
  LUT0/1 -> AddSub/1
  LUT1/1 -> AddSub/2
  LUT2/1 -> AddSub1/1
  LUT3/1 -> AddSub1/2
  AddSub1/1 -> AddSub2/2
  AddSub/1 -> AddSub2/1
  AddSub3/1 -> Out2/1
  Slice4/1 -> LUT4/1
  Slice7/1 -> LUT7/1
  Slice6/1 -> LUT6/1
  Slice5/1 -> LUT5/1
  LUT4/1 -> AddSub4/1
  LUT5/1 -> AddSub4/2
  LUT6/1 -> AddSub5/1
  LUT7/1 -> AddSub5/2
  AddSub5/1 -> AddSub6/2
  AddSub4/1 -> AddSub6/1
  AddSub2/1 -> AddSub3/1
  AddSub6/1 -> AddSub3/2

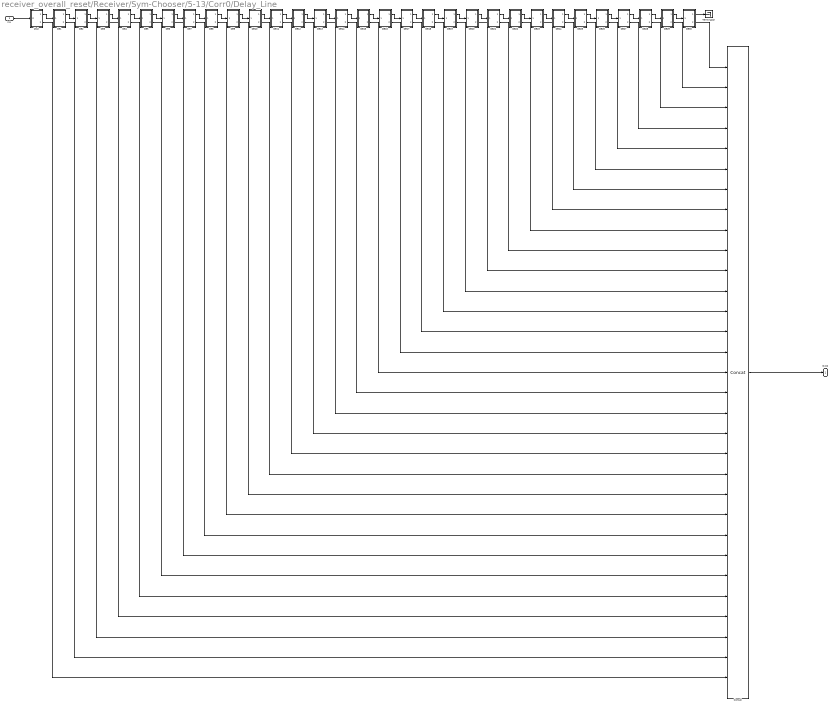
== system receiver_overall_reset/Receiver/Sym-Chooser/5-13/Corr0/Delay_Line ==
  In1 : Inport
  1to2 : Subsystem
  Concat : xbsIndex_r4/Concat  num_inputs=31  dbl_ovrd=off  block_type=concat
      settings: block_version=12.1
  DE1 : Subsystem
      mask Display: disp('z^{-1}','texmode','on')
  DE10 : Subsystem
      mask Display: disp('z^{-1}','texmode','on')
  DE11 : Subsystem
      mask Display: disp('z^{-1}','texmode','on')
  DE12 : Subsystem
      mask Display: disp('z^{-1}','texmode','on')
  DE13 : Subsystem
      mask Display: disp('z^{-1}','texmode','on')
  DE14 : Subsystem
      mask Display: disp('z^{-1}','texmode','on')
  DE15 : Subsystem
      mask Display: disp('z^{-1}','texmode','on')
  DE16 : Subsystem
      mask Display: disp('z^{-1}','texmode','on')
  DE17 : Subsystem
      mask Display: disp('z^{-1}','texmode','on')
  DE18 : Subsystem
      mask Display: disp('z^{-1}','texmode','on')
  DE19 : Subsystem
      mask Display: disp('z^{-1}','texmode','on')
  DE2 : Subsystem
      mask Display: disp('z^{-1}','texmode','on')
  DE20 : Subsystem
      mask Display: disp('z^{-1}','texmode','on')
  DE21 : Subsystem
      mask Display: disp('z^{-1}','texmode','on')
  DE22 : Subsystem
      mask Display: disp('z^{-1}','texmode','on')
  DE23 : Subsystem
      mask Display: disp('z^{-1}','texmode','on')
  DE24 : Subsystem
      mask Display: disp('z^{-1}','texmode','on')
  DE25 : Subsystem
      mask Display: disp('z^{-1}','texmode','on')
  DE26 : Subsystem
      mask Display: disp('z^{-1}','texmode','on')
  DE27 : Subsystem
      mask Display: disp('z^{-1}','texmode','on')
  DE28 : Subsystem
      mask Display: disp('z^{-1}','texmode','on')
  DE29 : Subsystem
      mask Display: disp('z^{-1}','texmode','on')
  DE3 : Subsystem
      mask Display: disp('z^{-1}','texmode','on')
  DE30 : Subsystem
      mask Display: disp('z^{-1}','texmode','on')
  DE4 : Subsystem
      mask Display: disp('z^{-1}','texmode','on')
  DE5 : Subsystem
      mask Display: disp('z^{-1}','texmode','on')
  DE6 : Subsystem
      mask Display: disp('z^{-1}','texmode','on')
  DE7 : Subsystem
      mask Display: disp('z^{-1}','texmode','on')
  DE8 : Subsystem
      mask Display: disp('z^{-1}','texmode','on')
  DE9 : Subsystem
      mask Display: disp('z^{-1}','texmode','on')
  Terminator : Terminator
  Out2 : Outport
  wires:
  Concat/1 -> Out2/1
  In1/1 -> 1to2/1(In)
  1to2/1(Out1) -> DE1/1(In1)
  DE30/1(Out1) -> Terminator/1
  1to2/2(Out2) -> Concat/31
  DE1/2(Out2) -> Concat/30
  DE2/2(Out2) -> Concat/29
  DE3/2(Out2) -> Concat/28
  DE4/2(Out2) -> Concat/27
  DE5/2(Out2) -> Concat/26
  DE6/2(Out2) -> Concat/25
  DE7/2(Out2) -> Concat/24
  DE8/2(Out2) -> Concat/23
  DE9/2(Out2) -> Concat/22
  DE10/2(Out2) -> Concat/21
  DE11/2(Out2) -> Concat/20
  DE12/2(Out2) -> Concat/19
  DE13/2(Out2) -> Concat/18
  DE14/2(Out2) -> Concat/17
  DE15/2(Out2) -> Concat/16
  DE16/2(Out2) -> Concat/15
  DE17/2(Out2) -> Concat/14
  DE18/2(Out2) -> Concat/13
  DE19/2(Out2) -> Concat/12
  DE20/2(Out2) -> Concat/11
  DE21/2(Out2) -> Concat/10
  DE22/2(Out2) -> Concat/9
  DE23/2(Out2) -> Concat/8
  DE24/2(Out2) -> Concat/7
  DE25/2(Out2) -> Concat/6
  DE26/2(Out2) -> Concat/5
  DE27/2(Out2) -> Concat/4
  DE28/2(Out2) -> Concat/3
  DE29/2(Out2) -> Concat/2
  DE30/2(Out2) -> Concat/1
  DE2/1(Out1) -> DE3/1(In1)
  DE3/1(Out1) -> DE4/1(In1)
  DE4/1(Out1) -> DE5/1(In1)
  DE5/1(Out1) -> DE6/1(In1)
  DE6/1(Out1) -> DE7/1(In1)
  DE7/1(Out1) -> DE8/1(In1)
  DE8/1(Out1) -> DE9/1(In1)
  DE9/1(Out1) -> DE10/1(In1)
  DE10/1(Out1) -> DE11/1(In1)
  DE11/1(Out1) -> DE12/1(In1)
  DE12/1(Out1) -> DE13/1(In1)
  DE13/1(Out1) -> DE14/1(In1)
  DE14/1(Out1) -> DE15/1(In1)
  DE15/1(Out1) -> DE16/1(In1)
  DE16/1(Out1) -> DE17/1(In1)
  DE17/1(Out1) -> DE18/1(In1)
  DE18/1(Out1) -> DE19/1(In1)
  DE19/1(Out1) -> DE20/1(In1)
  DE20/1(Out1) -> DE21/1(In1)
  DE21/1(Out1) -> DE22/1(In1)
  DE22/1(Out1) -> DE23/1(In1)
  DE23/1(Out1) -> DE24/1(In1)
  DE24/1(Out1) -> DE25/1(In1)
  DE25/1(Out1) -> DE26/1(In1)
  DE26/1(Out1) -> DE27/1(In1)
  DE27/1(Out1) -> DE28/1(In1)
  DE28/1(Out1) -> DE29/1(In1)
  DE29/1(Out1) -> DE30/1(In1)
  DE1/1(Out1) -> DE2/1(In1)

== system receiver_overall_reset/Receiver/Sym-Chooser/6-14/Corr0/Corr ==
  In1 : Inport
  AddSub{,1..6} (7 alike) : xbsIndex_r4/AddSub  mode=Addition  use_carryin=off  use_carryout=off  en=off  latency=0  precision=Full  arith_type=Unsigned  n_bits=16  bin_pt=14  quantization=Truncate  overflow=Wrap  dbl_ovrd=off  use_behavioral_HDL=off  hw_selection=Fabric  pipelined=off  block_type=addsub
      AddSub settings: xl_area=[2 0 0 3 0 0 0]  block_version=12.1
      AddSub1 settings: xl_area=[2 0 0 3 0 0 0]  block_version=12.1
      AddSub2 settings: xl_area=[3 0 0 4 0 0 0]  block_version=12.1
      AddSub3 settings: xl_area=[3 0 0 5 0 0 0]  block_version=12.1
      AddSub4 settings: xl_area=[2 0 0 3 0 0 0]  block_version=12.1
      AddSub5 settings: xl_area=[2 0 0 3 0 0 0]  block_version=12.1
      AddSub6 settings: xl_area=[3 0 0 4 0 0 0]  block_version=12.1
  LUT{0..7} (8 alike) : xbsIndex_r4/ROM  depth=16  initVector=[0,1,1,2,1,2,2,3,1,2,2,3,2,3,3,4]  distributed_mem=Distributed memory  rst=off  init_reg=0  en=off  latency=0  arith_type=Unsigned  n_bits=3  bin_pt=0  dbl_ovrd=off  optimize=Area  use_rpm=on  block_type=sprom
      settings: xl_area=[0 0 1 0 0 0 0]  block_version=12.1
  Slice0 : xbsIndex_r4/Slice  nbits=4  boolean_output=off  mode=Lower Bit Location + Width  bit1=0  base1=MSB of Input  bit0=0  base0=LSB of Input  dbl_ovrd=off  block_type=slice
      settings: block_version=12.1
  Slice1 : xbsIndex_r4/Slice  nbits=4  boolean_output=off  mode=Lower Bit Location + Width  bit1=-4  base1=MSB of Input  bit0=4  base0=LSB of Input  dbl_ovrd=off  block_type=slice
      settings: block_version=12.1
  Slice2 : xbsIndex_r4/Slice  nbits=4  boolean_output=off  mode=Lower Bit Location + Width  bit1=-8  base1=MSB of Input  bit0=8  base0=LSB of Input  dbl_ovrd=off  block_type=slice
      settings: block_version=12.1
  Slice3 : xbsIndex_r4/Slice  nbits=4  boolean_output=off  mode=Lower Bit Location + Width  bit1=-12  base1=MSB of Input  bit0=12  base0=LSB of Input  dbl_ovrd=off  block_type=slice
      settings: block_version=12.1
  Slice4 : xbsIndex_r4/Slice  nbits=4  boolean_output=off  mode=Lower Bit Location + Width  bit1=0  base1=LSB of Input  bit0=16  base0=LSB of Input  dbl_ovrd=off  block_type=slice
      settings: block_version=12.1
  Slice5 : xbsIndex_r4/Slice  nbits=4  boolean_output=off  mode=Lower Bit Location + Width  bit1=0  base1=LSB of Input  bit0=20  base0=LSB of Input  dbl_ovrd=off  block_type=slice
      settings: block_version=12.1
  Slice6 : xbsIndex_r4/Slice  nbits=4  boolean_output=off  mode=Lower Bit Location + Width  bit1=0  base1=LSB of Input  bit0=24  base0=LSB of Input  dbl_ovrd=off  block_type=slice
      settings: block_version=12.1
  Slice7 : xbsIndex_r4/Slice  nbits=4  boolean_output=off  mode=Lower Bit Location + Width  bit1=0  base1=LSB of Input  bit0=28  base0=LSB of Input  dbl_ovrd=off  block_type=slice
      settings: block_version=12.1
  Out2 : Outport
  wires:
  In1/1 -> Slice0/1, Slice1/1, Slice2/1, Slice7/1, Slice6/1, Slice3/1, Slice4/1, Slice5/1
  Slice0/1 -> LUT0/1
  Slice3/1 -> LUT3/1
  Slice2/1 -> LUT2/1
  Slice1/1 -> LUT1/1
  LUT0/1 -> AddSub/1
  LUT1/1 -> AddSub/2
  LUT2/1 -> AddSub1/1
  LUT3/1 -> AddSub1/2
  AddSub1/1 -> AddSub2/2
  AddSub/1 -> AddSub2/1
  AddSub3/1 -> Out2/1
  Slice4/1 -> LUT4/1
  Slice7/1 -> LUT7/1
  Slice6/1 -> LUT6/1
  Slice5/1 -> LUT5/1
  LUT4/1 -> AddSub4/1
  LUT5/1 -> AddSub4/2
  LUT6/1 -> AddSub5/1
  LUT7/1 -> AddSub5/2
  AddSub5/1 -> AddSub6/2
  AddSub4/1 -> AddSub6/1
  AddSub2/1 -> AddSub3/1
  AddSub6/1 -> AddSub3/2

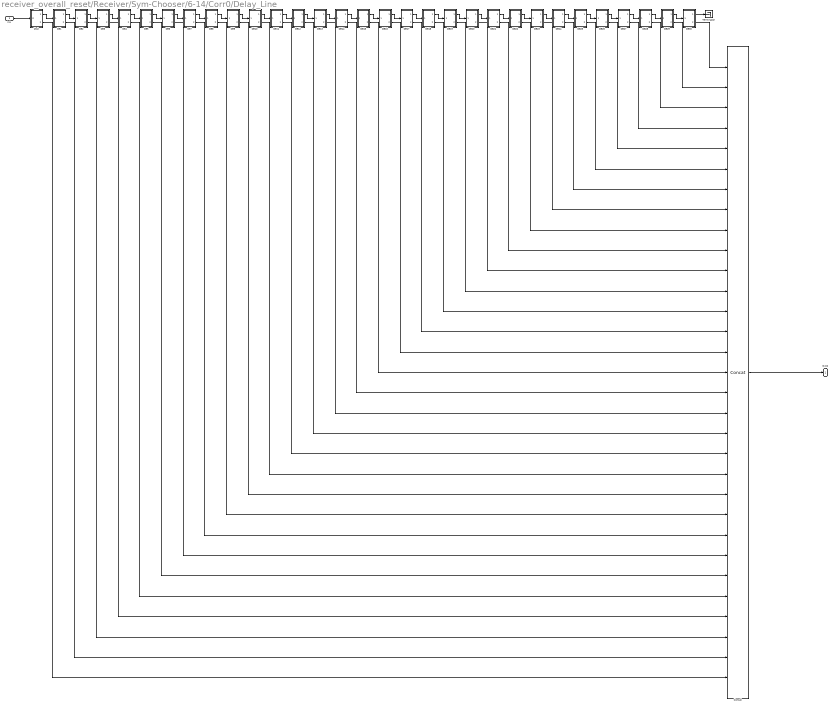
== system receiver_overall_reset/Receiver/Sym-Chooser/6-14/Corr0/Delay_Line ==
  In1 : Inport
  1to2 : Subsystem
  Concat : xbsIndex_r4/Concat  num_inputs=31  dbl_ovrd=off  block_type=concat
      settings: block_version=12.1
  DE1 : Subsystem
      mask Display: disp('z^{-1}','texmode','on')
  DE10 : Subsystem
      mask Display: disp('z^{-1}','texmode','on')
  DE11 : Subsystem
      mask Display: disp('z^{-1}','texmode','on')
  DE12 : Subsystem
      mask Display: disp('z^{-1}','texmode','on')
  DE13 : Subsystem
      mask Display: disp('z^{-1}','texmode','on')
  DE14 : Subsystem
      mask Display: disp('z^{-1}','texmode','on')
  DE15 : Subsystem
      mask Display: disp('z^{-1}','texmode','on')
  DE16 : Subsystem
      mask Display: disp('z^{-1}','texmode','on')
  DE17 : Subsystem
      mask Display: disp('z^{-1}','texmode','on')
  DE18 : Subsystem
      mask Display: disp('z^{-1}','texmode','on')
  DE19 : Subsystem
      mask Display: disp('z^{-1}','texmode','on')
  DE2 : Subsystem
      mask Display: disp('z^{-1}','texmode','on')
  DE20 : Subsystem
      mask Display: disp('z^{-1}','texmode','on')
  DE21 : Subsystem
      mask Display: disp('z^{-1}','texmode','on')
  DE22 : Subsystem
      mask Display: disp('z^{-1}','texmode','on')
  DE23 : Subsystem
      mask Display: disp('z^{-1}','texmode','on')
  DE24 : Subsystem
      mask Display: disp('z^{-1}','texmode','on')
  DE25 : Subsystem
      mask Display: disp('z^{-1}','texmode','on')
  DE26 : Subsystem
      mask Display: disp('z^{-1}','texmode','on')
  DE27 : Subsystem
      mask Display: disp('z^{-1}','texmode','on')
  DE28 : Subsystem
      mask Display: disp('z^{-1}','texmode','on')
  DE29 : Subsystem
      mask Display: disp('z^{-1}','texmode','on')
  DE3 : Subsystem
      mask Display: disp('z^{-1}','texmode','on')
  DE30 : Subsystem
      mask Display: disp('z^{-1}','texmode','on')
  DE4 : Subsystem
      mask Display: disp('z^{-1}','texmode','on')
  DE5 : Subsystem
      mask Display: disp('z^{-1}','texmode','on')
  DE6 : Subsystem
      mask Display: disp('z^{-1}','texmode','on')
  DE7 : Subsystem
      mask Display: disp('z^{-1}','texmode','on')
  DE8 : Subsystem
      mask Display: disp('z^{-1}','texmode','on')
  DE9 : Subsystem
      mask Display: disp('z^{-1}','texmode','on')
  Terminator : Terminator
  Out2 : Outport
  wires:
  Concat/1 -> Out2/1
  In1/1 -> 1to2/1(In)
  1to2/1(Out1) -> DE1/1(In1)
  DE30/1(Out1) -> Terminator/1
  1to2/2(Out2) -> Concat/31
  DE1/2(Out2) -> Concat/30
  DE2/2(Out2) -> Concat/29
  DE3/2(Out2) -> Concat/28
  DE4/2(Out2) -> Concat/27
  DE5/2(Out2) -> Concat/26
  DE6/2(Out2) -> Concat/25
  DE7/2(Out2) -> Concat/24
  DE8/2(Out2) -> Concat/23
  DE9/2(Out2) -> Concat/22
  DE10/2(Out2) -> Concat/21
  DE11/2(Out2) -> Concat/20
  DE12/2(Out2) -> Concat/19
  DE13/2(Out2) -> Concat/18
  DE14/2(Out2) -> Concat/17
  DE15/2(Out2) -> Concat/16
  DE16/2(Out2) -> Concat/15
  DE17/2(Out2) -> Concat/14
  DE18/2(Out2) -> Concat/13
  DE19/2(Out2) -> Concat/12
  DE20/2(Out2) -> Concat/11
  DE21/2(Out2) -> Concat/10
  DE22/2(Out2) -> Concat/9
  DE23/2(Out2) -> Concat/8
  DE24/2(Out2) -> Concat/7
  DE25/2(Out2) -> Concat/6
  DE26/2(Out2) -> Concat/5
  DE27/2(Out2) -> Concat/4
  DE28/2(Out2) -> Concat/3
  DE29/2(Out2) -> Concat/2
  DE30/2(Out2) -> Concat/1
  DE2/1(Out1) -> DE3/1(In1)
  DE3/1(Out1) -> DE4/1(In1)
  DE4/1(Out1) -> DE5/1(In1)
  DE5/1(Out1) -> DE6/1(In1)
  DE6/1(Out1) -> DE7/1(In1)
  DE7/1(Out1) -> DE8/1(In1)
  DE8/1(Out1) -> DE9/1(In1)
  DE9/1(Out1) -> DE10/1(In1)
  DE10/1(Out1) -> DE11/1(In1)
  DE11/1(Out1) -> DE12/1(In1)
  DE12/1(Out1) -> DE13/1(In1)
  DE13/1(Out1) -> DE14/1(In1)
  DE14/1(Out1) -> DE15/1(In1)
  DE15/1(Out1) -> DE16/1(In1)
  DE16/1(Out1) -> DE17/1(In1)
  DE17/1(Out1) -> DE18/1(In1)
  DE18/1(Out1) -> DE19/1(In1)
  DE19/1(Out1) -> DE20/1(In1)
  DE20/1(Out1) -> DE21/1(In1)
  DE21/1(Out1) -> DE22/1(In1)
  DE22/1(Out1) -> DE23/1(In1)
  DE23/1(Out1) -> DE24/1(In1)
  DE24/1(Out1) -> DE25/1(In1)
  DE25/1(Out1) -> DE26/1(In1)
  DE26/1(Out1) -> DE27/1(In1)
  DE27/1(Out1) -> DE28/1(In1)
  DE28/1(Out1) -> DE29/1(In1)
  DE29/1(Out1) -> DE30/1(In1)
  DE1/1(Out1) -> DE2/1(In1)

== system receiver_overall_reset/Receiver/Sym-Chooser/7-15/Corr0/Corr ==
  In1 : Inport
  AddSub{,1..6} (7 alike) : xbsIndex_r4/AddSub  mode=Addition  use_carryin=off  use_carryout=off  en=off  latency=0  precision=Full  arith_type=Unsigned  n_bits=16  bin_pt=14  quantization=Truncate  overflow=Wrap  dbl_ovrd=off  use_behavioral_HDL=off  hw_selection=Fabric  pipelined=off  block_type=addsub
      AddSub settings: xl_area=[2 0 0 3 0 0 0]  block_version=12.1
      AddSub1 settings: xl_area=[2 0 0 3 0 0 0]  block_version=12.1
      AddSub2 settings: xl_area=[3 0 0 4 0 0 0]  block_version=12.1
      AddSub3 settings: xl_area=[3 0 0 5 0 0 0]  block_version=12.1
      AddSub4 settings: xl_area=[2 0 0 3 0 0 0]  block_version=12.1
      AddSub5 settings: xl_area=[2 0 0 3 0 0 0]  block_version=12.1
      AddSub6 settings: xl_area=[3 0 0 4 0 0 0]  block_version=12.1
  LUT{0..7} (8 alike) : xbsIndex_r4/ROM  depth=16  initVector=[0,1,1,2,1,2,2,3,1,2,2,3,2,3,3,4]  distributed_mem=Distributed memory  rst=off  init_reg=0  en=off  latency=0  arith_type=Unsigned  n_bits=3  bin_pt=0  dbl_ovrd=off  optimize=Area  use_rpm=on  block_type=sprom
      settings: xl_area=[0 0 1 0 0 0 0]  block_version=12.1
  Slice0 : xbsIndex_r4/Slice  nbits=4  boolean_output=off  mode=Lower Bit Location + Width  bit1=0  base1=MSB of Input  bit0=0  base0=LSB of Input  dbl_ovrd=off  block_type=slice
      settings: block_version=12.1
  Slice1 : xbsIndex_r4/Slice  nbits=4  boolean_output=off  mode=Lower Bit Location + Width  bit1=-4  base1=MSB of Input  bit0=4  base0=LSB of Input  dbl_ovrd=off  block_type=slice
      settings: block_version=12.1
  Slice2 : xbsIndex_r4/Slice  nbits=4  boolean_output=off  mode=Lower Bit Location + Width  bit1=-8  base1=MSB of Input  bit0=8  base0=LSB of Input  dbl_ovrd=off  block_type=slice
      settings: block_version=12.1
  Slice3 : xbsIndex_r4/Slice  nbits=4  boolean_output=off  mode=Lower Bit Location + Width  bit1=-12  base1=MSB of Input  bit0=12  base0=LSB of Input  dbl_ovrd=off  block_type=slice
      settings: block_version=12.1
  Slice4 : xbsIndex_r4/Slice  nbits=4  boolean_output=off  mode=Lower Bit Location + Width  bit1=0  base1=LSB of Input  bit0=16  base0=LSB of Input  dbl_ovrd=off  block_type=slice
      settings: block_version=12.1
  Slice5 : xbsIndex_r4/Slice  nbits=4  boolean_output=off  mode=Lower Bit Location + Width  bit1=0  base1=LSB of Input  bit0=20  base0=LSB of Input  dbl_ovrd=off  block_type=slice
      settings: block_version=12.1
  Slice6 : xbsIndex_r4/Slice  nbits=4  boolean_output=off  mode=Lower Bit Location + Width  bit1=0  base1=LSB of Input  bit0=24  base0=LSB of Input  dbl_ovrd=off  block_type=slice
      settings: block_version=12.1
  Slice7 : xbsIndex_r4/Slice  nbits=4  boolean_output=off  mode=Lower Bit Location + Width  bit1=0  base1=LSB of Input  bit0=28  base0=LSB of Input  dbl_ovrd=off  block_type=slice
      settings: block_version=12.1
  Out2 : Outport
  wires:
  In1/1 -> Slice0/1, Slice1/1, Slice2/1, Slice7/1, Slice6/1, Slice3/1, Slice4/1, Slice5/1
  Slice0/1 -> LUT0/1
  Slice3/1 -> LUT3/1
  Slice2/1 -> LUT2/1
  Slice1/1 -> LUT1/1
  LUT0/1 -> AddSub/1
  LUT1/1 -> AddSub/2
  LUT2/1 -> AddSub1/1
  LUT3/1 -> AddSub1/2
  AddSub1/1 -> AddSub2/2
  AddSub/1 -> AddSub2/1
  AddSub3/1 -> Out2/1
  Slice4/1 -> LUT4/1
  Slice7/1 -> LUT7/1
  Slice6/1 -> LUT6/1
  Slice5/1 -> LUT5/1
  LUT4/1 -> AddSub4/1
  LUT5/1 -> AddSub4/2
  LUT6/1 -> AddSub5/1
  LUT7/1 -> AddSub5/2
  AddSub5/1 -> AddSub6/2
  AddSub4/1 -> AddSub6/1
  AddSub2/1 -> AddSub3/1
  AddSub6/1 -> AddSub3/2

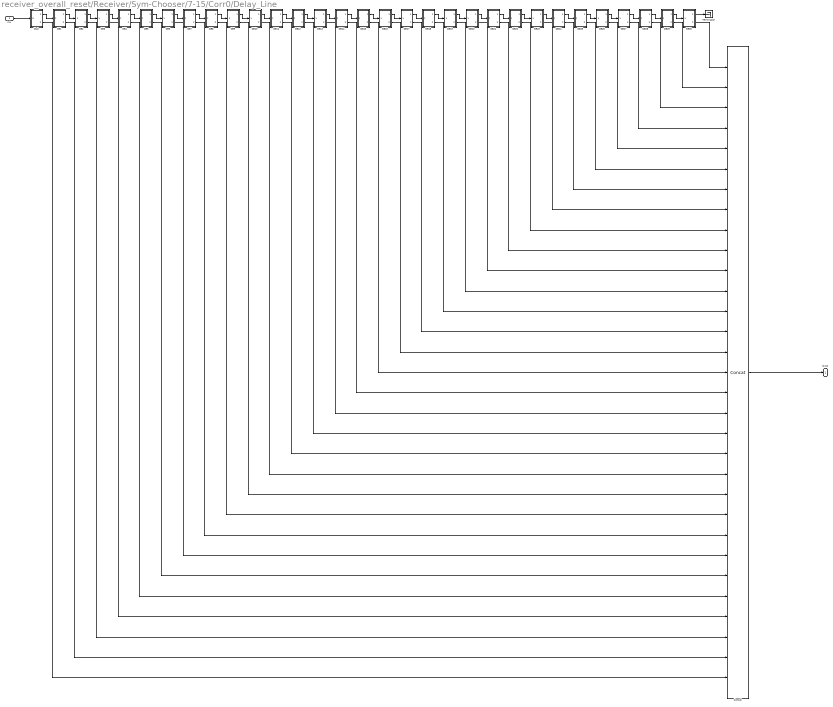
== system receiver_overall_reset/Receiver/Sym-Chooser/7-15/Corr0/Delay_Line ==
  In1 : Inport
  1to2 : Subsystem
  Concat : xbsIndex_r4/Concat  num_inputs=31  dbl_ovrd=off  block_type=concat
      settings: block_version=12.1
  DE1 : Subsystem
      mask Display: disp('z^{-1}','texmode','on')
  DE10 : Subsystem
      mask Display: disp('z^{-1}','texmode','on')
  DE11 : Subsystem
      mask Display: disp('z^{-1}','texmode','on')
  DE12 : Subsystem
      mask Display: disp('z^{-1}','texmode','on')
  DE13 : Subsystem
      mask Display: disp('z^{-1}','texmode','on')
  DE14 : Subsystem
      mask Display: disp('z^{-1}','texmode','on')
  DE15 : Subsystem
      mask Display: disp('z^{-1}','texmode','on')
  DE16 : Subsystem
      mask Display: disp('z^{-1}','texmode','on')
  DE17 : Subsystem
      mask Display: disp('z^{-1}','texmode','on')
  DE18 : Subsystem
      mask Display: disp('z^{-1}','texmode','on')
  DE19 : Subsystem
      mask Display: disp('z^{-1}','texmode','on')
  DE2 : Subsystem
      mask Display: disp('z^{-1}','texmode','on')
  DE20 : Subsystem
      mask Display: disp('z^{-1}','texmode','on')
  DE21 : Subsystem
      mask Display: disp('z^{-1}','texmode','on')
  DE22 : Subsystem
      mask Display: disp('z^{-1}','texmode','on')
  DE23 : Subsystem
      mask Display: disp('z^{-1}','texmode','on')
  DE24 : Subsystem
      mask Display: disp('z^{-1}','texmode','on')
  DE25 : Subsystem
      mask Display: disp('z^{-1}','texmode','on')
  DE26 : Subsystem
      mask Display: disp('z^{-1}','texmode','on')
  DE27 : Subsystem
      mask Display: disp('z^{-1}','texmode','on')
  DE28 : Subsystem
      mask Display: disp('z^{-1}','texmode','on')
  DE29 : Subsystem
      mask Display: disp('z^{-1}','texmode','on')
  DE3 : Subsystem
      mask Display: disp('z^{-1}','texmode','on')
  DE30 : Subsystem
      mask Display: disp('z^{-1}','texmode','on')
  DE4 : Subsystem
      mask Display: disp('z^{-1}','texmode','on')
  DE5 : Subsystem
      mask Display: disp('z^{-1}','texmode','on')
  DE6 : Subsystem
      mask Display: disp('z^{-1}','texmode','on')
  DE7 : Subsystem
      mask Display: disp('z^{-1}','texmode','on')
  DE8 : Subsystem
      mask Display: disp('z^{-1}','texmode','on')
  DE9 : Subsystem
      mask Display: disp('z^{-1}','texmode','on')
  Terminator : Terminator
  Out2 : Outport
  wires:
  Concat/1 -> Out2/1
  In1/1 -> 1to2/1(In)
  1to2/1(Out1) -> DE1/1(In1)
  DE30/1(Out1) -> Terminator/1
  1to2/2(Out2) -> Concat/31
  DE1/2(Out2) -> Concat/30
  DE2/2(Out2) -> Concat/29
  DE3/2(Out2) -> Concat/28
  DE4/2(Out2) -> Concat/27
  DE5/2(Out2) -> Concat/26
  DE6/2(Out2) -> Concat/25
  DE7/2(Out2) -> Concat/24
  DE8/2(Out2) -> Concat/23
  DE9/2(Out2) -> Concat/22
  DE10/2(Out2) -> Concat/21
  DE11/2(Out2) -> Concat/20
  DE12/2(Out2) -> Concat/19
  DE13/2(Out2) -> Concat/18
  DE14/2(Out2) -> Concat/17
  DE15/2(Out2) -> Concat/16
  DE16/2(Out2) -> Concat/15
  DE17/2(Out2) -> Concat/14
  DE18/2(Out2) -> Concat/13
  DE19/2(Out2) -> Concat/12
  DE20/2(Out2) -> Concat/11
  DE21/2(Out2) -> Concat/10
  DE22/2(Out2) -> Concat/9
  DE23/2(Out2) -> Concat/8
  DE24/2(Out2) -> Concat/7
  DE25/2(Out2) -> Concat/6
  DE26/2(Out2) -> Concat/5
  DE27/2(Out2) -> Concat/4
  DE28/2(Out2) -> Concat/3
  DE29/2(Out2) -> Concat/2
  DE30/2(Out2) -> Concat/1
  DE2/1(Out1) -> DE3/1(In1)
  DE3/1(Out1) -> DE4/1(In1)
  DE4/1(Out1) -> DE5/1(In1)
  DE5/1(Out1) -> DE6/1(In1)
  DE6/1(Out1) -> DE7/1(In1)
  DE7/1(Out1) -> DE8/1(In1)
  DE8/1(Out1) -> DE9/1(In1)
  DE9/1(Out1) -> DE10/1(In1)
  DE10/1(Out1) -> DE11/1(In1)
  DE11/1(Out1) -> DE12/1(In1)
  DE12/1(Out1) -> DE13/1(In1)
  DE13/1(Out1) -> DE14/1(In1)
  DE14/1(Out1) -> DE15/1(In1)
  DE15/1(Out1) -> DE16/1(In1)
  DE16/1(Out1) -> DE17/1(In1)
  DE17/1(Out1) -> DE18/1(In1)
  DE18/1(Out1) -> DE19/1(In1)
  DE19/1(Out1) -> DE20/1(In1)
  DE20/1(Out1) -> DE21/1(In1)
  DE21/1(Out1) -> DE22/1(In1)
  DE22/1(Out1) -> DE23/1(In1)
  DE23/1(Out1) -> DE24/1(In1)
  DE24/1(Out1) -> DE25/1(In1)
  DE25/1(Out1) -> DE26/1(In1)
  DE26/1(Out1) -> DE27/1(In1)
  DE27/1(Out1) -> DE28/1(In1)
  DE28/1(Out1) -> DE29/1(In1)
  DE29/1(Out1) -> DE30/1(In1)
  DE1/1(Out1) -> DE2/1(In1)

== system receiver_overall_reset/Receiver/Sym-Clk/Corr/Delay_Line/1to2 ==
  In : Inport  OutDataType=fixdt(1, 16)  OutScaling=2^0
  Out1 : Outport  OutDataType=fixdt(1, 16)  OutScaling=2^0
  Out2 : Outport  Port=2  OutDataType=fixdt(1, 16)  OutScaling=2^0
  wires:
  In/1 -> Out1/1, Out2/1

== system receiver_overall_reset/Receiver/Sym-Clk/Corr/Delay_Line/DE1 ==
  In1 : Inport
  1to2 : Subsystem
  DE : xbsIndex_r4/Delay  en=off  latency=1  dbl_ovrd=off  reg_retiming=off  block_type=delay
      settings: xl_area=[1 1 0 0 0 0 0]  block_version=12.1
  Out1 : Outport
  Out2 : Outport  Port=2
  wires:
  DE/1 -> 1to2/1(In)
  In1/1 -> DE/1
  1to2/1(Out1) -> Out1/1
  1to2/2(Out2) -> Out2/1

== system receiver_overall_reset/Receiver/Sym-Clk/Corr/Delay_Line/DE10 ==
  In1 : Inport
  1to2 : Subsystem
  DE : xbsIndex_r4/Delay  en=off  latency=1  dbl_ovrd=off  reg_retiming=off  block_type=delay
      settings: xl_area=[1 1 0 0 0 0 0]  block_version=12.1
  Out1 : Outport
  Out2 : Outport  Port=2
  wires:
  1to2/2(Out2) -> Out2/1
  1to2/1(Out1) -> Out1/1
  In1/1 -> DE/1
  DE/1 -> 1to2/1(In)

== system receiver_overall_reset/Receiver/Sym-Clk/Corr/Delay_Line/DE11 ==
  In1 : Inport
  1to2 : Subsystem
  DE : xbsIndex_r4/Delay  en=off  latency=1  dbl_ovrd=off  reg_retiming=off  block_type=delay
      settings: xl_area=[1 1 0 0 0 0 0]  block_version=12.1
  Out1 : Outport
  Out2 : Outport  Port=2
  wires:
  1to2/2(Out2) -> Out2/1
  1to2/1(Out1) -> Out1/1
  In1/1 -> DE/1
  DE/1 -> 1to2/1(In)

== system receiver_overall_reset/Receiver/Sym-Clk/Corr/Delay_Line/DE12 ==
  In1 : Inport
  1to2 : Subsystem
  DE : xbsIndex_r4/Delay  en=off  latency=1  dbl_ovrd=off  reg_retiming=off  block_type=delay
      settings: xl_area=[1 1 0 0 0 0 0]  block_version=12.1
  Out1 : Outport
  Out2 : Outport  Port=2
  wires:
  1to2/2(Out2) -> Out2/1
  1to2/1(Out1) -> Out1/1
  In1/1 -> DE/1
  DE/1 -> 1to2/1(In)

== system receiver_overall_reset/Receiver/Sym-Clk/Corr/Delay_Line/DE13 ==
  In1 : Inport
  1to2 : Subsystem
  DE : xbsIndex_r4/Delay  en=off  latency=1  dbl_ovrd=off  reg_retiming=off  block_type=delay
      settings: xl_area=[1 1 0 0 0 0 0]  block_version=12.1
  Out1 : Outport
  Out2 : Outport  Port=2
  wires:
  1to2/2(Out2) -> Out2/1
  1to2/1(Out1) -> Out1/1
  In1/1 -> DE/1
  DE/1 -> 1to2/1(In)

== system receiver_overall_reset/Receiver/Sym-Clk/Corr/Delay_Line/DE14 ==
  In1 : Inport
  1to2 : Subsystem
  DE : xbsIndex_r4/Delay  en=off  latency=1  dbl_ovrd=off  reg_retiming=off  block_type=delay
      settings: xl_area=[1 1 0 0 0 0 0]  block_version=12.1
  Out1 : Outport
  Out2 : Outport  Port=2
  wires:
  1to2/2(Out2) -> Out2/1
  1to2/1(Out1) -> Out1/1
  In1/1 -> DE/1
  DE/1 -> 1to2/1(In)

== system receiver_overall_reset/Receiver/Sym-Clk/Corr/Delay_Line/DE15 ==
  In1 : Inport
  1to2 : Subsystem
  DE : xbsIndex_r4/Delay  en=off  latency=1  dbl_ovrd=off  reg_retiming=off  block_type=delay
      settings: xl_area=[1 1 0 0 0 0 0]  block_version=12.1
  Out1 : Outport
  Out2 : Outport  Port=2
  wires:
  1to2/2(Out2) -> Out2/1
  1to2/1(Out1) -> Out1/1
  In1/1 -> DE/1
  DE/1 -> 1to2/1(In)
